simulink model "FullModel"  (R2020a)
settings: Solver=VariableStepAuto  StartTime=0.0  StopTime=100  RelTol=1e-3
settings Model: Creator=micha  LastModifiedBy=micha

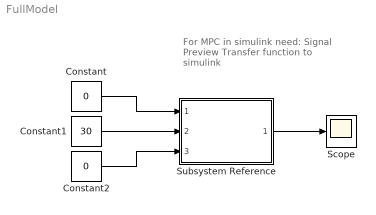
== system FullModel ==
  note: For MPC in simulink need:
      | 	Signal Preview
      | 	Transfer function to simulink
  Constant : Constant  Value=0
  Constant1 : Constant  Value=30
  Constant2 : Constant  Value=0
  Scope : Scope
  Subsystem Reference : Subsystem  ReferencedSubsystem=plantDynamics
  wires:
  Constant/1 -> Subsystem Reference/1
  Constant1/1 -> Subsystem Reference/2
  Constant2/1 -> Subsystem Reference/3
  Subsystem Reference/1 -> Scope/1
